simulink model "Pendulum_Project_R2023a"  (R2023b)
settings: Solver=VariableStepAuto  StartTime=0.0  StopTime=15  MaxStep=1e-3  RelTol=1e-3
settings Model: Creator=hp  LastModifiedBy=hp

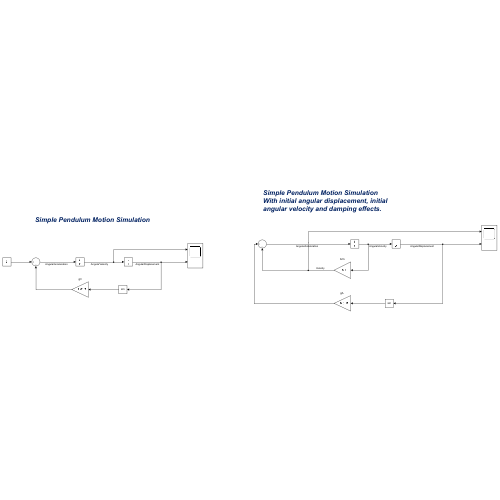
[thumbnail: Simulink's stored preview of the top-level diagram]
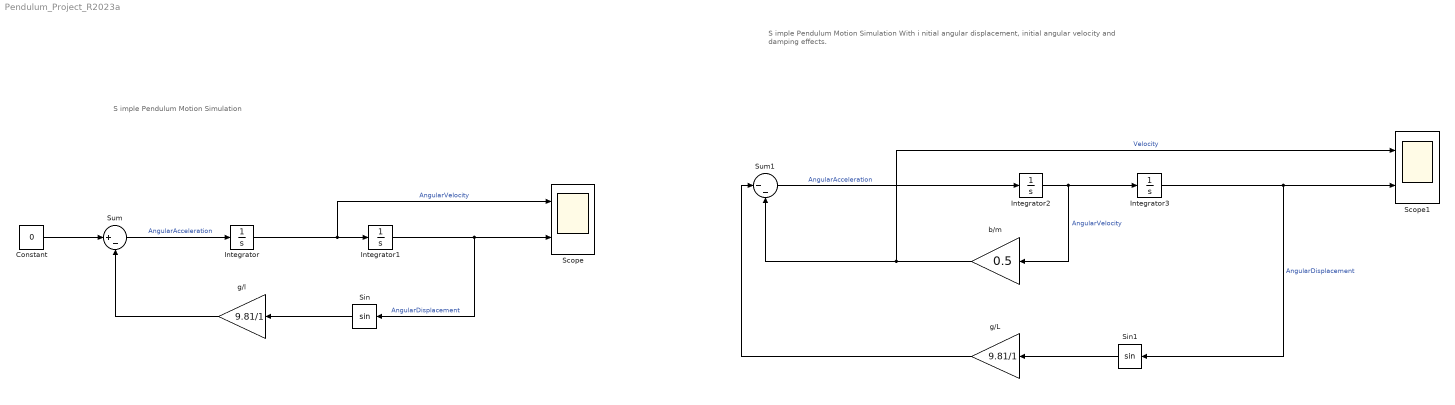
== system Pendulum_Project_R2023a ==
  note: S imple Pendulum Motion Simulation
      | With i nitial angular displacement, initial angular velocity and damping effects.
  note: S imple Pendulum Motion Simulation
  Constant : Constant  Value=0
  Integrator : Integrator
  Integrator1 : Integrator  InitialCondition=0.5
  Integrator2 : Integrator  InitialCondition=0.1
  Integrator3 : Integrator  InitialCondition=0.5
  Scope : Scope  NumInputPorts=2
  Scope1 : Scope  NumInputPorts=2
  Sin : Trigonometry
  Sin1 : Trigonometry
  Sum : Sum  Inputs=|+-
  Sum1 : Sum  Inputs=|--
  b/m : Gain  Gain=0.5
  g/L : Gain  Gain=9.81/1
  g/l : Gain  Gain=9.81/1
  wires:
  Constant/1 -> Sum/1
  Sum/1 -> Integrator/1  "AngularAcceleration"
  Integrator/1 -> Scope/1, Integrator1/1  "AngularVelocity"
  g/l/1 -> Sum/2
  Sin/1 -> g/l/1
  Integrator1/1 -> Sin/1, Scope/2  "AngularDisplacement"
  Integrator3/1 -> Sin1/1, Scope1/2  "AngularDisplacement"
  Sin1/1 -> g/L/1
  Integrator2/1 -> b/m/1, Integrator3/1  "AngularVelocity"
  Sum1/1 -> Integrator2/1  "AngularAcceleration"
  g/L/1 -> Sum1/1
  b/m/1 -> Scope1/1, Sum1/2  "Velocity"
